simulink model "ex_direct_lookup_table_4d_table_is_input"  (R2017b)
settings: Solver=FixedStepDiscrete  StartTime=0.0  StopTime=10.0  FixedStep=0.100000  RelTol=1e-3  EnableMultiTasking=on
PreLoadFcn:
  | a = reshape(1:2800, [4 5 20 7]);
settings Model: Creator=The MathWorks, Inc.  LastModifiedBy=hbourbou
settings DataIOCC: LimitDataPoints=on
settings OptimizationCC: ExpressionDepthLimit=2147483647  LifeSpan=inf
settings DebuggingCC: UnderspecifiedInitializationDetection=Classic  MergeDetectMultiDrivingBlocksExec=none  SolverPrmCheckMsg=warning  FcnCallInpInsideContextMsg=warning  StateNameClashWarn=warning  StrictBusMsg=Warning  SFUnexpectedBacktrackingDiag=warning  SFNoUnconditionalDefaultTransitionDiag=warning  SFExecutionAtInitializationDiag=none
settings HardwareCC: ProdBitPerPointer=32  ProdBitPerSizeT=32  ProdBitPerPtrDiffT=32  ProdLargestAtomicFloat=None  ProdIntDivRoundTo=Undefined  ProdEndianess=Unspecified  ProdWordSize=32  ProdHWDeviceType=32-bit Generic
settings ModelReferenceCC: PropagateSignalLabelsOutOfModel=off
settings RTWCC: Description=Generic Real-Time Target
settings CodeAppCC: StateflowObjectComments=on
settings GRTTargetCC: TargetLangStandard=C89/C90 (ANSI)  GeneratePreprocessorConditionals=Disable all  CombineOutputUpdateFcns=off  GRTInterface=on
settings ConfigComp: CovMetricSettings=dw  CovHtmlReporting=on  CovSaveCumulativeToWorkspaceVar=on  CovSaveSingleToWorkspaceVar=on  CovExternalEMLEnable=off

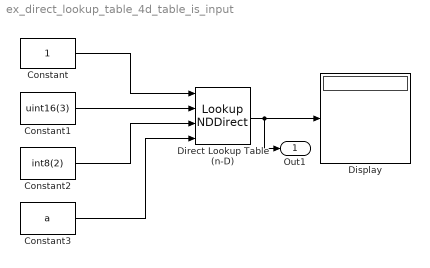
== system ex_direct_lookup_table_4d_table_is_input ==
  Constant : Constant
  Constant1 : Constant  Value=uint16(3)
  Constant2 : Constant  Value=int8(2)
  Constant3 : Constant  Value=a  OutDataTypeStr=double
  Direct Lookup Table (n-D) : LookupNDDirect  NumberOfTableDimensions=4  InputsSelectThisObjectFromTable=Column  TableIsInput=on
  Display : Display
  Out1 : Outport
  wires:
  Constant/1 -> Direct Lookup Table (n-D)/1
  Constant1/1 -> Direct Lookup Table (n-D)/2
  Constant2/1 -> Direct Lookup Table (n-D)/3
  Direct Lookup Table (n-D)/1 -> Out1/1, Display/1
  Constant3/1 -> Direct Lookup Table (n-D)/4
